simulink model "pv_environment"  (R2024b)
settings: Solver=ode1  StartTime=0.0  StopTime=60  FixedStep=1e-5  MaxStep=1e-5  RelTol=1e-3
undefined symbols (not defined in the file or in its folder): algo_id
libraries: spsSeriesRLCBranchLib x4, spsCurrentMeasurementLib x2, spsVoltageMeasurementLib x2, spsDiodeLib x1, spsMosfetLib x1, spsPVArrayLib x1, spsPWMGeneratorDCDCLib x1, spspowerguiLib x1
settings Model: Creator=DELL 7450  LastModifiedBy=hp

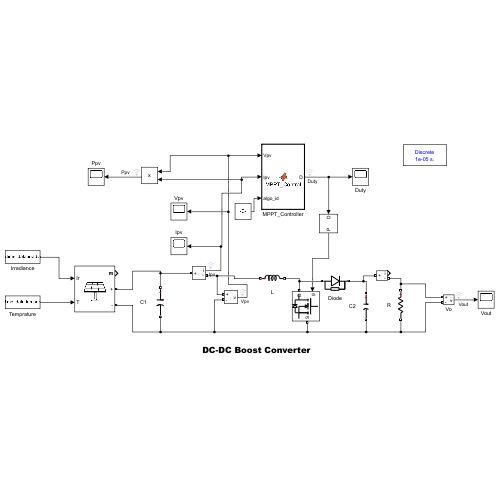
[thumbnail: Simulink's stored preview of the top-level diagram]
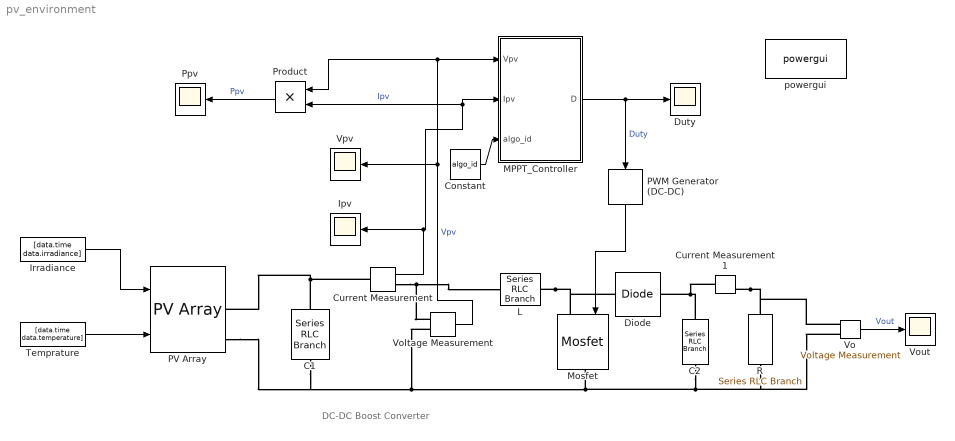
== system pv_environment ==
  note: DC-DC Boost Converter
  C1 : spsSeriesRLCBranchLib/Series RLC Branch  LConnTagsString=__new0  RConnTagsString=__new0  BranchType=C  Resistance=1  Inductance=1e-3  SetiL0=off  InitialCurrent=0  Capacitance=14.397e-6  Setx0=off  InitialVoltage=0  Measurements=None
  C2 : spsSeriesRLCBranchLib/Series RLC Branch  LConnTagsString=__new0  RConnTagsString=__new0  BranchType=C  Resistance=1  Inductance=1e-3  SetiL0=off  InitialCurrent=0  Capacitance=4700e-5  Setx0=off  InitialVoltage=0  Measurements=None
  Constant : Constant  Value=algo_id
  Current Measurement : spsCurrentMeasurementLib/Current Measurement  PhasorSimulation=off  OutputType=Complex  PSBequivalent=0
  Current Measurement1 : spsCurrentMeasurementLib/Current Measurement  PhasorSimulation=off  OutputType=Complex  PSBequivalent=0
  Diode : spsDiodeLib/Diode  Ron=0.001  Lon=0  Vf=0.8  IC=0  UseSnubber=0  Rs=500  Cs=250e-9  Measurements=off
  Duty : Scope
  Ipv : Scope
  Irradiance : FromWorkspace  VariableName="[data.time  data.irradiance]"  SampleTime=0.001  OutputAfterFinalValue=Holding final value
  L : spsSeriesRLCBranchLib/Series RLC Branch  LConnTagsString=__new0  RConnTagsString=__new0  BranchType=L  Resistance=1  Inductance=20e-3  SetiL0=off  InitialCurrent=0  Capacitance=1e-6  Setx0=off  InitialVoltage=0  Measurements=None
  MPPT_Controller : MATLAB Function  TreatAsAtomicUnit=on
  Mosfet : spsMosfetLib/Mosfet  Ron=0.1  Lon=0  Rd=0.01  Vfd=0  IC=0  Rs=1e5  Cs=inf  Measurements=off
  PV Array : spsPVArrayLib/PV Array  Npar=1  Nser=1  PlotType=array @ 1000 W/m2 & specified temperatures  S_vec="[ 1000  500  100 ]"  Temp_C_vec="[ 45 25  ]"  ModuleName=User-defined  PlotWhenSelected=off  Pm=540.15  Ncell=144  Voc=49.50  Isc=13.81  Vm=41.55  Im=13.00  beta_Voc_pc=-0.36099  alpha_Isc_pc=0.102  beta_Voc=-0.17869  alpha_Isc=0.014086  IL=13.8809  I0=5.1615e-10  nI=0.55756  Rsh=195.3922  Rs=0.13175  RobustModel=off  RobustCellTemperature=313.3991  BAL=on  Tc=1e-6  Tfilter=5e-5
  PWM Generator (DC-DC) : spsPWMGeneratorDCDCLib/PWM Generator (DC-DC)  Fsw=10e3  Ts=1e-5
  Ppv : Scope
  Product : Product
  R : spsSeriesRLCBranchLib/Series RLC Branch  LConnTagsString=__new0  RConnTagsString=__new0  BranchType=R  Resistance=20  Inductance=1e-3  SetiL0=off  InitialCurrent=0  Capacitance=1e-6  Setx0=off  InitialVoltage=0  Measurements=None
  Temprature : FromWorkspace  VariableName="[data.time  data.temperature]"  SampleTime=0.001  OutputAfterFinalValue=Holding final value
  Vo : spsVoltageMeasurementLib/Voltage Measurement  PhasorSimulation=off  OutputType=Complex  PSBequivalent=0
  Voltage Measurement : spsVoltageMeasurementLib/Voltage Measurement  PhasorSimulation=off  OutputType=Complex  PSBequivalent=0
  Vout : Scope
  Vpv : Scope
  powergui : spspowerguiLib/powergui  Priority=1  SimulationMode=Discrete  SampleTime=1e-5  frequency=60  Iterations=50  frequencyindice=0  Pbase=100e6  ErrMax=1e-4  UnitsV=kV  UnitsW=MW  buscounter=0  FunctionMessages=off  echomessages=off  EnableUseOfTLC=off  CurrentSourceSwitches=off  DisableSnubberDevices=off  DisableRonSwitches=off  DisableVfSwitches=off  DisplayEquations=off  AutomaticDiscreteSolvers=off  SolverType=Tustin/Backward Euler (TBE)  Interpol=off  ExternalGateDelay=off  methode=off  Ts=100  x0status=blocks  SPID=on  SwTol=0  HookPort=off  NonlinearTolerance=1e-4  nMaxIteration=100  ContinueOnMaxIteration=off  RestoreLinks=warning  ResistiveCurrentMeasurement=off  Frange=[0:2:500]  Ylog=off  Xlog=on  ShowGrid=off  save=off  variable=ZData  structure=0  ZoomFFT=off  StartTime=0.0  cycles=1  DisplayStyle=1  fundamental=60  FreqAxis=off  MaxFrequency=1000  frequencyindicesteady=1  RmsSteady=1  display=off
  wires:
  Vo/1 -> Vout/1  "Vout"
  Current Measurement/1 -> Ipv/1, MPPT_Controller/2(Ipv), Product/2  "Ipv"
  Voltage Measurement/1 -> Vpv/1, Product/1, MPPT_Controller/1(Vpv)  "Vpv"
  MPPT_Controller/1(D) -> PWM Generator (DC-DC)/1, Duty/1  "Duty"
  PWM Generator (DC-DC)/1 -> Mosfet/1
  Irradiance/1 -> PV Array/1
  Temprature/1 -> PV Array/2
  Product/1 -> Ppv/1  "Ppv"
  Constant/1 -> MPPT_Controller/3(algo_id)
  connections:
  C1/RConn1 -- PV Array/RConn2 -- Voltage Measurement/LConn2 -- R/RConn1 -- Vo/LConn2 -- C2/RConn1 -- Mosfet/RConn1
  Current Measurement/LConn1 -- C1/LConn1 -- PV Array/RConn1
  C2/LConn1 -- Current Measurement1/LConn1 -- Diode/RConn1
  Current Measurement1/RConn1 -- R/LConn1 -- Vo/LConn1
  L/RConn1 -- Mosfet/LConn1 -- Diode/LConn1
  Current Measurement/RConn1 -- Voltage Measurement/LConn1 -- L/LConn1

== matlab function pv_environment/MPPT_Controller ==
  settings: updateMethod=DISCRETE
  data: Vpv input; D output; Ipv input; algo_id input
function D = MPPT_Control(Vpv, Ipv, algo_id)

%#codegen

switch algo_id
    
    case 1
        D = mppt_PO(Vpv, Ipv);
        
    case 2
        D = mppt_IncCond(Vpv, Ipv);
        
    case 3
        D = mppt_SMC(Vpv, Ipv);
        
    case 4
        D = mppt_RCC(Vpv, Ipv);
        
    case 5
        D = mppt_FSB(Vpv, Ipv);
        
    case 6
        D = mppt_FLC(Vpv, Ipv);
        
    case 7
        D = mppt_ANN(Vpv, Ipv);
        
    case 8
        D = mppt_PSO(Vpv, Ipv);
        
    case 9
        D = mppt_GA(Vpv, Ipv);
        
    case 10
        D = mppt_GWO(Vpv, Ipv);
        
    otherwise
        D = 0.5;
end

end
